simulink model "bh_DDR_component_model"  (R2019b)
settings: Solver=ode45  StartTime=0.0  StopTime=120  RelTol=1e-5  EnableMultiTasking=on
undefined symbols (not defined in the file): veh
libraries: simulink_extras x2
settings Model: Creator=sriramn  LastModifiedBy=Pierce
settings SolverCC: ZeroCrossAlgorithm=Adaptive
settings DataIOCC: LimitDataPoints=on  SaveFormat=Array  ReturnWorkspaceOutputs=off
settings OptimizationCC: LifeSpan=inf
settings DebuggingCC: AlgebraicLoopMsg=error  SolverPrmCheckMsg=warning  AllowSymbolicDim=off  SFUnexpectedBacktrackingDiag=warning  SFNoUnconditionalDefaultTransitionDiag=warning  SFExecutionAtInitializationDiag=none  ArithmeticOperatorsInVariantConditions=warning
settings HardwareCC: ProdBitPerPointer=32  ProdBitPerSizeT=32  ProdBitPerPtrDiffT=32  ProdLargestAtomicFloat=None  ProdIntDivRoundTo=Undefined  ProdEndianess=Unspecified  ProdWordSize=32  ProdHWDeviceType=32-bit Generic
settings ModelReferenceCC: PropagateSignalLabelsOutOfModel=off
settings SFSimCC: SimUseLocalCustomCode=off  CustomCodeUndefinedFunction=UseInterfaceOnly
settings RTWCC: RTWUseLocalCustomCode=off
settings CodeAppCC: StateflowObjectComments=on
settings GRTTargetCC: TargetLangStandard=C89/C90 (ANSI)  GeneratePreprocessorConditionals=Disable all
settings ConfigComp: CovMetricSettings=dw  CovHtmlReporting=on  CovSaveCumulativeToWorkspaceVar=on  CovSaveSingleToWorkspaceVar=on  CovExternalEMLEnable=off  CovSFcnEnable=off
settings SimscapeCC: SimscapeNormalizeSystem=off
settings ConfigurationSet: Description=SimMechanics 2G
settings ExplorerConfigSet: InternalSimMechanicsExplorerSettings="<ExplorerConfiguration><canonicalview>planar_xy</canonicalview><AnimationSetting><BasePlaybackSpeed>1.0</BasePlaybackSpeed><PlaybackSpeedFactor>1.0</PlaybackSpeedFactor></AnimationSetting><TilePanel><TileInfo><Tiles Columns=\"1\" Count=\"1\" Rows=\"1\"><Column Left=\"2\" Weight=\"1\"/><Column Left=\"1628\"/><Row Top=\"2\" Weight=\"1\"/><Row Top=\"1072\"/><Tile Height=\"1\" Width=\"1\" X=\"0\" Y=\"0\"/></Tiles></TileInfo><SceneInfo><SceneViewer><BGColor><R>0.60000002384185791</R><G>0.60000002384185791</G><B>0.60000002384185791</B></BGColor><Camera><Position><X>0.22951840878551699</X><Y>0.32651610611526627</Y><Z>-0.27215421354393321</Z></Position><Center><X>-0.15775714411666431</X><Y>-0.15462825985839526</Y><Z>0.065702552916005602</Z></Center><Up><X>-0.56030137557930915</X><Y>0.72817587161684794</Y><Z>0.39474329445726858</Z></Up><Left>-0.21481383955700509</Left><Right>0.21481383955700509</Right><Bottom>-0.27569784609469139</Bottom><Top>0.27569784609469139</Top></Camera></SceneViewer></SceneInfo></TilePanel></ExplorerConfiguration>"

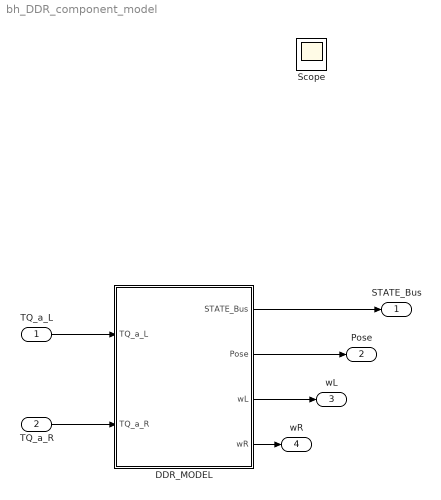
== system bh_DDR_component_model ==
  TQ_a_L : Inport
  TQ_a_R : Inport  Port=2
  DDR_MODEL : Subsystem  mask(EOM for differential drive robot){L=veh.L_half_axle, d=veh.d, m=veh.mass, I_veh=veh.Inertia, r=veh.wheel.r, m_w=veh.wheel.mass, I_w=veh.wheel.I, bR=veh.wheel.bR, bL=veh.wheel.bL, v_Cx_init=veh.states.init_vel_B_Cx, theta0_degs=0, theta0_dot_degs_per_sec=veh.states.init_theta_vel_deg, xy_G_init=[2,2]}
      mask prompts: L "Axle HALF length (L) separating wheels  (m)"; d "the offset (d) of Cg from axle (m)"; m "Total Vehicle mass (m) in (kg)"; I_veh "Total Vehicle Inertia (I_veh) in (kg.m^2)"; r "Radius (r) of driving wheels (m)"; m_w "Wheel mass (m_w) in (kg)"; I_w "Wheel and local shaft Inertia (Iw) in (kg.m^2)"; bR "RIGHT shaft viscous dampng (bR) in (N.m.sec/rad)"; bL "LEFT shaft viscous dampng (bR) in (N.m.sec/rad)"; v_Cx_init "Initial velocity vCx in the BODY  frame (m/sec)"; theta0_degs "Initial Theta position (degs)"; theta0_dot_degs_per_sec "Initial Theta velocity (degs/sec)"; xy_G_init "Initial (x,y) position in the {G}-frame (m)"
      mask help: Dynamic Model for a differential Drive robot.
      mask DialogControl Container10 Prompt: GEOMETRY
      mask DialogControl Container9 Prompt: INERTIA
      mask DialogControl Container12 Prompt: WHEELS
      mask DialogControl Control5 Prompt: We'll assume that the mass and inertia of the two wheels are the same, but we will let each wheel have different viscous damping.
      mask DialogControl Container6 Prompt: STATES
      mask Display: image(imread('bh_pics_veh_01.JPG'));
  STATE_Bus : Outport  OutDataTypeStr=Bus: BUS_DDR_state
  Pose : Outport  Port=2
  wL : Outport  Port=3
  wR : Outport  Port=4
  Scope : Scope
  wires:
  DDR_MODEL/1(STATE_Bus) -> STATE_Bus/1
  DDR_MODEL/2(Pose) -> Pose/1
  DDR_MODEL/3(wL) -> wL/1
  DDR_MODEL/4(wR) -> wR/1
  TQ_a_L/1 -> DDR_MODEL/1(TQ_a_L)
  TQ_a_R/1 -> DDR_MODEL/2(TQ_a_R)

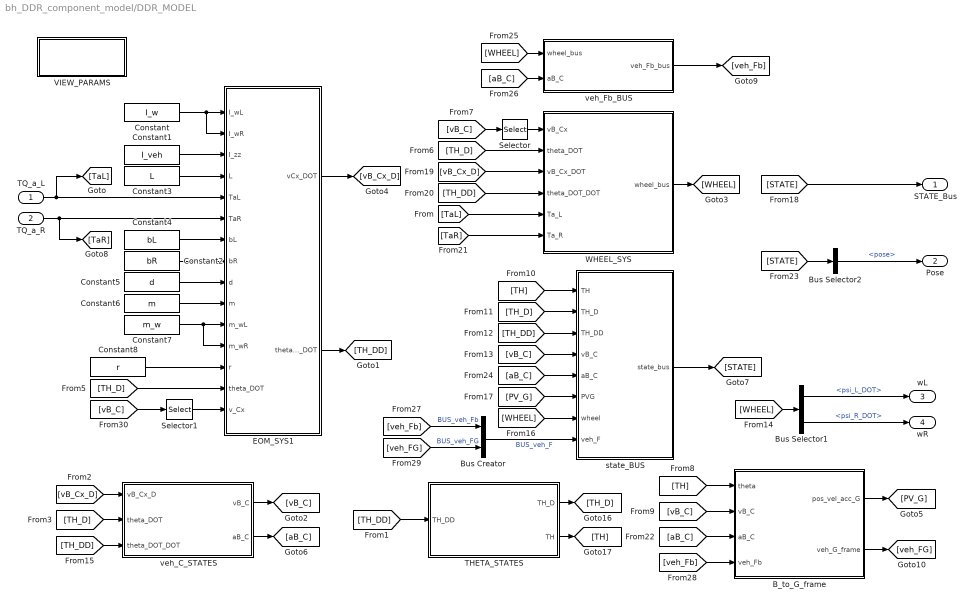
== system bh_DDR_component_model/DDR_MODEL ==
  TQ_a_L : Inport
  TQ_a_R : Inport  Port=2
  B_to_G_frame : Subsystem
  Bus Creator : BusCreator  Inputs=2
  Bus Selector1 : BusSelector  OutputSignals=BUS_wheel_vel.psi_L_DOT,BUS_wheel_vel.psi_R_DOT
  Bus Selector2 : BusSelector  OutputSignals=pose
  Constant : Constant  Value=I_w
  Constant1 : Constant  Value=I_veh
  Constant2 : Constant  Value=bR
  Constant3 : Constant  Value=L
  Constant4 : Constant  Value=bL
  Constant5 : Constant  Value=d
  Constant6 : Constant  Value=m
  Constant7 : Constant  Value=m_w
  Constant8 : Constant  Value=r
  EOM_SYS1 : MATLAB Function  TreatAsAtomicUnit=on
  Selector : Selector  InputPortWidth=2  IndexOptions=Index vector (dialog)  Indices=1  OutputSizes=1
  Selector1 : Selector  InputPortWidth=2  IndexOptions=Index vector (dialog)  Indices=1  OutputSizes=1
  THETA_STATES : Subsystem
  VIEW_PARAMS : Subsystem
  WHEEL_SYS : Subsystem
  state_BUS : Subsystem
  veh_C_STATES : Subsystem
  veh_Fb_BUS : Subsystem
  STATE_Bus : Outport
  Pose : Outport  Port=2
  wL : Outport  Port=3
  wR : Outport  Port=4
  wires:
  Constant1/1 -> EOM_SYS1/3(I_zz)
  Constant3/1 -> EOM_SYS1/4(L)
  Constant2/1 -> EOM_SYS1/8(bR)
  Constant4/1 -> EOM_SYS1/7(bL)
  Constant5/1 -> EOM_SYS1/9(d)
  Constant6/1 -> EOM_SYS1/10(m)
  Constant8/1 -> EOM_SYS1/13(r)
  TQ_a_L/1 -> EOM_SYS1/5(TaL), [TaL]
  TQ_a_R/1 -> EOM_SYS1/6(TaR), [TaR]
  [TH_DD] -> THETA_STATES/1(TH_DD)
  THETA_STATES/1(TH_D) -> [TH_D]
  THETA_STATES/2(TH) -> [TH]
  EOM_SYS1/2(theta_DOT_DOT) -> [TH_DD]
  [vB_Cx_D] -> veh_C_STATES/1(vB_Cx_D)
  EOM_SYS1/1(vCx_DOT) -> [vB_Cx_D]
  veh_C_STATES/1(vB_C) -> [vB_C]
  [TH_D] -> EOM_SYS1/14(theta_DOT)
  Selector1/1 -> EOM_SYS1/15(v_Cx)
  [vB_C] -> Selector/1
  [vB_C] -> B_to_G_frame/2(vB_C)
  [TH] -> B_to_G_frame/1(theta)
  B_to_G_frame/1(pos_vel_acc_G) -> [PV_G]
  [TH] -> state_BUS/1(TH)
  [TH_D] -> state_BUS/2(TH_D)
  [TH_DD] -> state_BUS/3(TH_DD)
  [WHEEL] -> state_BUS/7(wheel)
  [PV_G] -> state_BUS/6(PVG)
  state_BUS/1(state_bus) -> [STATE]
  [STATE] -> STATE_Bus/1
  [TH_D] -> WHEEL_SYS/2(theta_DOT)
  [vB_Cx_D] -> WHEEL_SYS/3(vB_Cx_DOT)
  [TH_DD] -> WHEEL_SYS/4(theta_DOT_DOT)
  WHEEL_SYS/1(wheel_bus) -> [WHEEL]
  [TaL] -> WHEEL_SYS/5(Ta_L)
  [TaR] -> WHEEL_SYS/6(Ta_R)
  [TH_D] -> veh_C_STATES/2(theta_DOT)
  Selector/1 -> WHEEL_SYS/1(vB_Cx)
  [vB_C] -> state_BUS/4(vB_C)
  [aB_C] -> state_BUS/5(aB_C)
  [TH_DD] -> veh_C_STATES/3(theta_DOT_DOT)
  veh_C_STATES/2(aB_C) -> [aB_C]
  [aB_C] -> B_to_G_frame/3(aB_C)
  [WHEEL] -> Bus Selector1/1
  Bus Selector1/1 -> wL/1  "<psi_L_DOT>"
  Bus Selector1/2 -> wR/1  "<psi_R_DOT>"
  [STATE] -> Bus Selector2/1
  Bus Selector2/1 -> Pose/1  "<pose>"
  [aB_C] -> veh_Fb_BUS/2(aB_C)
  [WHEEL] -> veh_Fb_BUS/1(wheel_bus)
  veh_Fb_BUS/1(veh_Fb_bus) -> [veh_Fb]
  [veh_Fb] -> B_to_G_frame/4(veh_Fb)
  B_to_G_frame/2(veh_G_frame) -> [veh_FG]
  [veh_Fb] -> Bus Creator/1  "BUS_veh_Fb"
  [veh_FG] -> Bus Creator/2  "BUS_veh_FG"
  Bus Creator/1 -> state_BUS/8(veh_F)  "BUS_veh_F"
  Constant/1 -> EOM_SYS1/2(I_wR), EOM_SYS1/1(I_wL)
  Constant7/1 -> EOM_SYS1/12(m_wR), EOM_SYS1/11(m_wL)
  [vB_C] -> Selector1/1

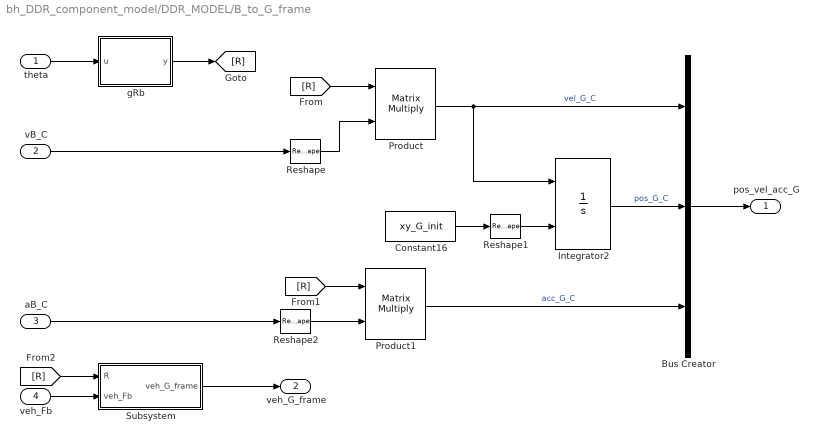
== system bh_DDR_component_model/DDR_MODEL/B_to_G_frame ==
  theta : Inport
  vB_C : Inport  Port=2
  aB_C : Inport  Port=3
  veh_Fb : Inport  Port=4
  Bus Creator : BusCreator  Inputs=3
  Constant16 : Constant  Value=xy_G_init
  Integrator2 : Integrator  InitialConditionSource=external
  Product : Product  Multiplication=Matrix(*)
  Product1 : Product  Multiplication=Matrix(*)
  Reshape : Reshape
  Reshape1 : Reshape
  Reshape2 : Reshape
  Subsystem : Subsystem
  gRb : MATLAB Function  TreatAsAtomicUnit=on
  pos_vel_acc_G : Outport
  veh_G_frame : Outport  Port=2
  wires:
  theta/1 -> gRb/1(u)
  Reshape/1 -> Product/2
  Product/1 -> Integrator2/1, Bus Creator/1  "vel_G_C"
  Constant16/1 -> Reshape1/1
  Integrator2/1 -> Bus Creator/2  "pos_G_C"
  Reshape1/1 -> Integrator2/2
  Bus Creator/1 -> pos_vel_acc_G/1
  vB_C/1 -> Reshape/1
  gRb/1(y) -> [R]
  [R] -> Product/1
  aB_C/1 -> Reshape2/1
  Reshape2/1 -> Product1/2
  [R] -> Product1/1
  Product1/1 -> Bus Creator/3  "acc_G_C"
  [R] -> Subsystem/1(R)
  veh_Fb/1 -> Subsystem/2(veh_Fb)
  Subsystem/1(veh_G_frame) -> veh_G_frame/1

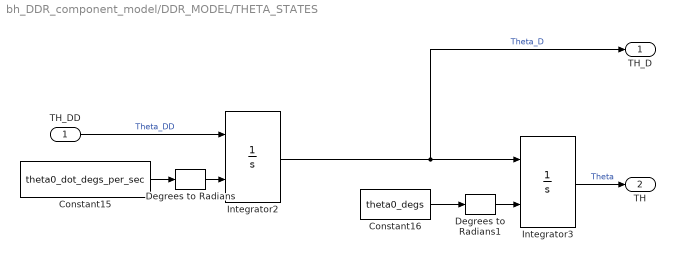
== system bh_DDR_component_model/DDR_MODEL/THETA_STATES ==
  TH_DD : Inport
  Constant15 : Constant  Value=theta0_dot_degs_per_sec
  Constant16 : Constant  Value=theta0_degs
  Degrees to Radians : simulink_extras/Transformations/Degrees to Radians
  Degrees to Radians1 : simulink_extras/Transformations/Degrees to Radians
  Integrator2 : Integrator  InitialConditionSource=external
  Integrator3 : Integrator  InitialConditionSource=external
  TH_D : Outport
  TH : Outport  Port=2
  wires:
  TH_DD/1 -> Integrator2/1  "Theta_DD"
  Integrator3/1 -> TH/1  "Theta"
  Integrator2/1 -> TH_D/1, Integrator3/1  "Theta_D"
  Degrees to Radians/1 -> Integrator2/2
  Degrees to Radians1/1 -> Integrator3/2
  Constant16/1 -> Degrees to Radians1/1
  Constant15/1 -> Degrees to Radians/1

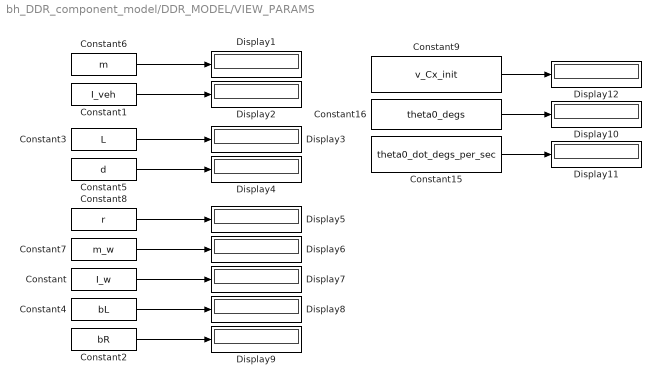
== system bh_DDR_component_model/DDR_MODEL/VIEW_PARAMS ==
  Constant : Constant  Value=I_w
  Constant1 : Constant  Value=I_veh
  Constant15 : Constant  Value=theta0_dot_degs_per_sec
  Constant16 : Constant  Value=theta0_degs
  Constant2 : Constant  Value=bR
  Constant3 : Constant  Value=L
  Constant4 : Constant  Value=bL
  Constant5 : Constant  Value=d
  Constant6 : Constant  Value=m
  Constant7 : Constant  Value=m_w
  Constant8 : Constant  Value=r
  Constant9 : Constant  Value=v_Cx_init
  Display{1..12} (12 alike) : Display
  wires:
  Constant6/1 -> Display1/1
  Constant1/1 -> Display2/1
  Constant5/1 -> Display4/1
  Constant3/1 -> Display3/1
  Constant7/1 -> Display6/1
  Constant8/1 -> Display5/1
  Constant/1 -> Display7/1
  Constant4/1 -> Display8/1
  Constant2/1 -> Display9/1
  Constant9/1 -> Display12/1
  Constant16/1 -> Display10/1
  Constant15/1 -> Display11/1

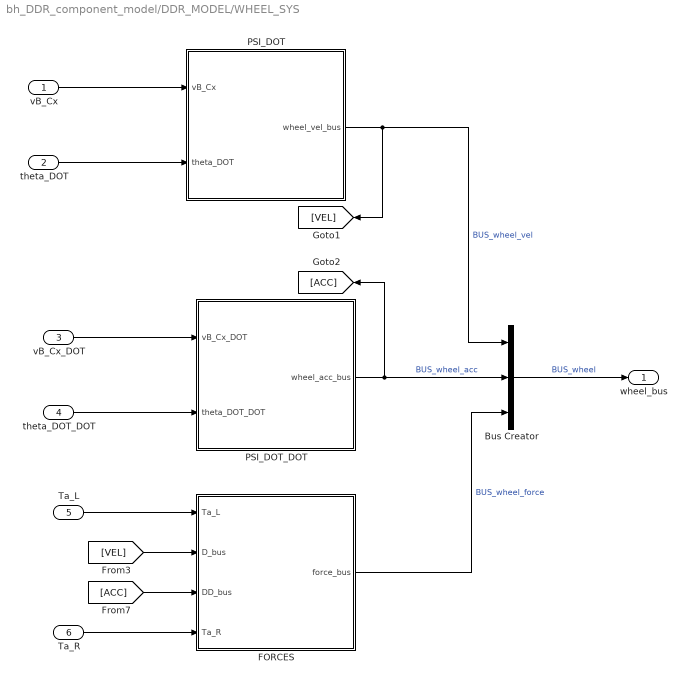
== system bh_DDR_component_model/DDR_MODEL/WHEEL_SYS ==
  vB_Cx : Inport
  theta_DOT : Inport  Port=2
  vB_Cx_DOT : Inport  Port=3
  theta_DOT_DOT : Inport  Port=4
  Ta_L : Inport  Port=5
  Ta_R : Inport  Port=6
  Bus Creator : BusCreator  Inputs=3
  FORCES : Subsystem
  PSI_DOT : Subsystem
  PSI_DOT_DOT : Subsystem
  wheel_bus : Outport
  wires:
  theta_DOT_DOT/1 -> PSI_DOT_DOT/2(theta_DOT_DOT)
  vB_Cx_DOT/1 -> PSI_DOT_DOT/1(vB_Cx_DOT)
  theta_DOT/1 -> PSI_DOT/2(theta_DOT)
  vB_Cx/1 -> PSI_DOT/1(vB_Cx)
  Bus Creator/1 -> wheel_bus/1  "BUS_wheel"
  PSI_DOT/1(wheel_vel_bus) -> [VEL], Bus Creator/1  "BUS_wheel_vel"
  PSI_DOT_DOT/1(wheel_acc_bus) -> Bus Creator/2, [ACC]  "BUS_wheel_acc"
  Ta_R/1 -> FORCES/4(Ta_R)
  Ta_L/1 -> FORCES/1(Ta_L)
  [ACC] -> FORCES/3(DD_bus)
  [VEL] -> FORCES/2(D_bus)
  FORCES/1(force_bus) -> Bus Creator/3  "BUS_wheel_force"

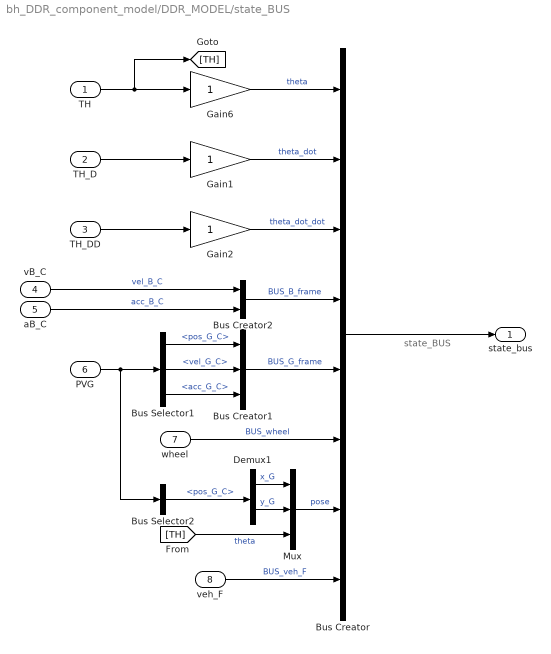
== system bh_DDR_component_model/DDR_MODEL/state_BUS ==
  note: state_BUS
  TH : Inport
  TH_D : Inport  Port=2
  TH_DD : Inport  Port=3
  vB_C : Inport  Port=4
  aB_C : Inport  Port=5
  PVG : Inport  Port=6
  wheel : Inport  Port=7
  veh_F : Inport  Port=8
  Bus Creator : BusCreator  Inputs=8
  Bus Creator1 : BusCreator  Inputs=3
  Bus Creator2 : BusCreator  Inputs=2
  Bus Selector1 : BusSelector  OutputSignals=pos_G_C,vel_G_C,acc_G_C
  Bus Selector2 : BusSelector  OutputSignals=pos_G_C
  Demux1 : Demux  Outputs=2
  Gain1 : Gain
  Gain2 : Gain
  Gain6 : Gain
  Mux : Mux  Inputs=3
  state_bus : Outport
  wires:
  Bus Creator/1 -> state_bus/1
  TH/1 -> [TH], Gain6/1
  TH_D/1 -> Gain1/1
  Gain6/1 -> Bus Creator/1  "theta"
  Gain1/1 -> Bus Creator/2  "theta_dot"
  TH_DD/1 -> Gain2/1
  Gain2/1 -> Bus Creator/3  "theta_dot_dot"
  vB_C/1 -> Bus Creator2/1  "vel_B_C"
  aB_C/1 -> Bus Creator2/2  "acc_B_C"
  PVG/1 -> Bus Selector2/1, Bus Selector1/1
  Bus Creator1/1 -> Bus Creator/5  "BUS_G_frame"
  wheel/1 -> Bus Creator/6  "BUS_wheel"
  Bus Creator2/1 -> Bus Creator/4  "BUS_B_frame"
  Bus Selector1/3 -> Bus Creator1/3  "<acc_G_C>"
  Bus Selector1/1 -> Bus Creator1/1  "<pos_G_C>"
  Bus Selector1/2 -> Bus Creator1/2  "<vel_G_C>"
  Mux/1 -> Bus Creator/7  "pose"
  Demux1/2 -> Mux/2  "y_G"
  Demux1/1 -> Mux/1  "x_G"
  [TH] -> Mux/3  "theta"
  Bus Selector2/1 -> Demux1/1  "<pos_G_C>"
  veh_F/1 -> Bus Creator/8  "BUS_veh_F"

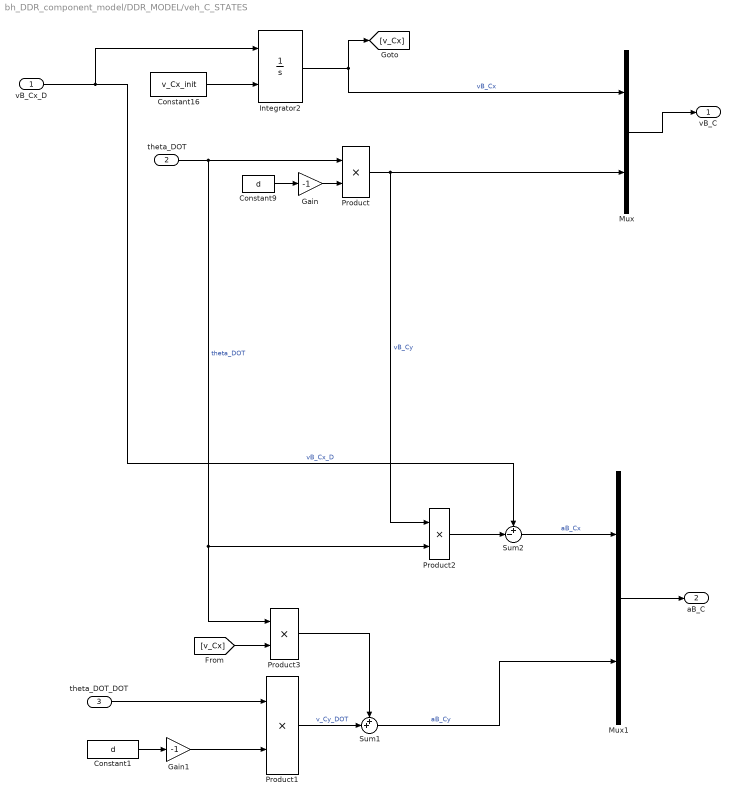
== system bh_DDR_component_model/DDR_MODEL/veh_C_STATES ==
  vB_Cx_D : Inport
  theta_DOT : Inport  Port=2
  theta_DOT_DOT : Inport  Port=3
  Constant1 : Constant  Value=d
  Constant16 : Constant  Value=v_Cx_init
  Constant9 : Constant  Value=d
  Gain : Gain  Gain=-1
  Gain1 : Gain  Gain=-1
  Integrator2 : Integrator  InitialConditionSource=external
  Mux : Mux  Inputs=2
  Mux1 : Mux  Inputs=2
  Product{,1..3} (4 alike) : Product
  Sum1 : Sum  Inputs=++|
  Sum2 : Sum  Inputs=+-|
  vB_C : Outport
  aB_C : Outport  Port=2
  wires:
  vB_Cx_D/1 -> Sum2/1, Integrator2/1  "vB_Cx_D"
  Constant16/1 -> Integrator2/2
  Integrator2/1 -> [v_Cx], Mux/1  "vB_Cx"
  theta_DOT/1 -> Product/1, Product3/1, Product2/2  "theta_DOT"
  Gain/1 -> Product/2
  Constant9/1 -> Gain/1
  Product/1 -> Product2/1, Mux/2  "vB_Cy"
  Mux/1 -> vB_C/1
  theta_DOT_DOT/1 -> Product1/1
  Gain1/1 -> Product1/2
  Constant1/1 -> Gain1/1
  Sum1/1 -> Mux1/2  "aB_Cy"
  Product2/1 -> Sum2/2
  Sum2/1 -> Mux1/1  "aB_Cx"
  Mux1/1 -> aB_C/1
  Product1/1 -> Sum1/2  "v_Cy_DOT"
  [v_Cx] -> Product3/2
  Product3/1 -> Sum1/1

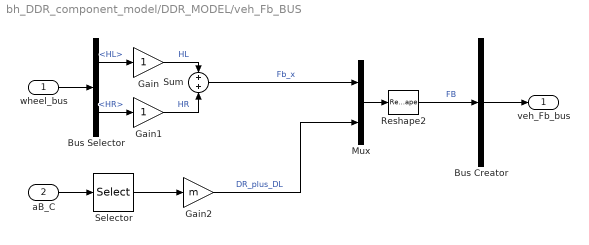
== system bh_DDR_component_model/DDR_MODEL/veh_Fb_BUS ==
  wheel_bus : Inport
  aB_C : Inport  Port=2
  Bus Creator : BusCreator  Inputs=1
  Bus Selector : BusSelector  OutputSignals=BUS_wheel_force.HL,BUS_wheel_force.HR
  Gain : Gain
  Gain1 : Gain
  Gain2 : Gain  Gain=m
  Mux : Mux  Inputs=2
  Reshape2 : Reshape
  Selector : Selector  InputPortWidth=2  IndexOptions=Index vector (dialog)  Indices=2  OutputSizes=1
  Sum : Sum  Inputs=+|+
  veh_Fb_bus : Outport
  wires:
  wheel_bus/1 -> Bus Selector/1
  Bus Selector/1 -> Gain/1  "<HL>"
  Bus Selector/2 -> Gain1/1  "<HR>"
  Gain/1 -> Sum/1  "HL"
  Gain1/1 -> Sum/2  "HR"
  Reshape2/1 -> Bus Creator/1  "FB"
  aB_C/1 -> Selector/1
  Selector/1 -> Gain2/1
  Sum/1 -> Mux/1  "Fb_x"
  Gain2/1 -> Mux/2  "DR_plus_DL"
  Mux/1 -> Reshape2/1
  Bus Creator/1 -> veh_Fb_bus/1

== system bh_DDR_component_model/DDR_MODEL/B_to_G_frame/Subsystem ==
  R : Inport
  veh_Fb : Inport  Port=2
  Bus Creator : BusCreator  Inputs=1
  Bus Selector : BusSelector  OutputSignals=FB
  Product1 : Product  Multiplication=Matrix(*)
  Reshape2 : Reshape
  veh_G_frame : Outport
  wires:
  Bus Selector/1 -> Reshape2/1  "<FB>"
  Reshape2/1 -> Product1/2
  R/1 -> Product1/1
  veh_Fb/1 -> Bus Selector/1
  Product1/1 -> Bus Creator/1  "FG"
  Bus Creator/1 -> veh_G_frame/1

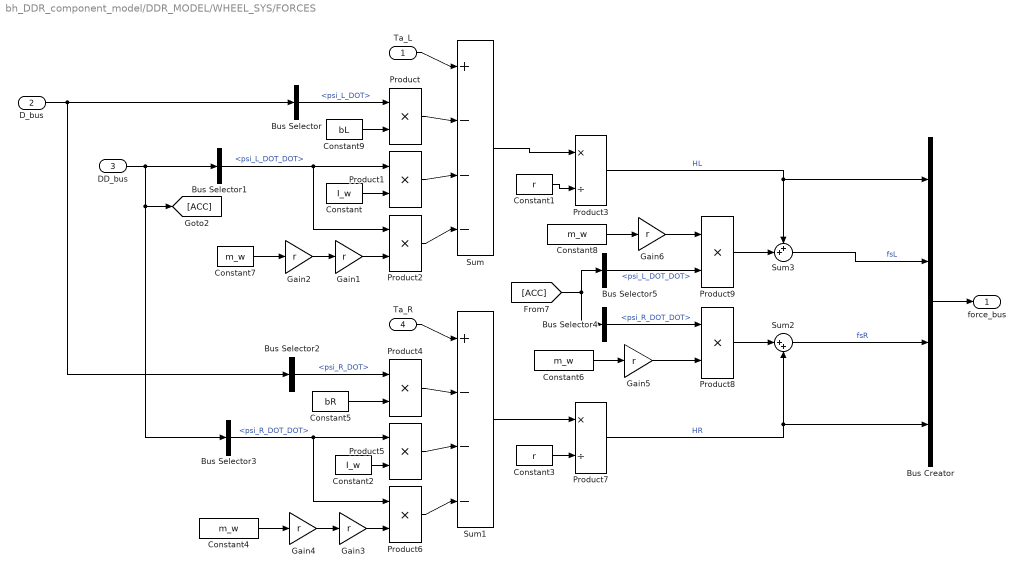
== system bh_DDR_component_model/DDR_MODEL/WHEEL_SYS/FORCES ==
  Ta_L : Inport
  D_bus : Inport  Port=2
  DD_bus : Inport  Port=3
  Ta_R : Inport  Port=4
  Bus Creator : BusCreator  Inputs=4
  Bus Selector : BusSelector  OutputSignals=psi_L_DOT
  Bus Selector1 : BusSelector  OutputSignals=psi_L_DOT_DOT
  Bus Selector2 : BusSelector  OutputSignals=psi_R_DOT
  Bus Selector3 : BusSelector  OutputSignals=psi_R_DOT_DOT
  Bus Selector4 : BusSelector  OutputSignals=psi_R_DOT_DOT
  Bus Selector5 : BusSelector  OutputSignals=psi_L_DOT_DOT
  Constant : Constant  Value=I_w
  Constant1 : Constant  Value=r
  Constant2 : Constant  Value=I_w
  Constant3 : Constant  Value=r
  Constant{4,6..8} (4 alike) : Constant  Value=m_w
  Constant5 : Constant  Value=bR
  Constant9 : Constant  Value=bL
  Gain{1..6} (6 alike) : Gain  Gain=r
  Product{,1..2,4..6,8..9} (8 alike) : Product
  Product3 : Product  Inputs=*/
  Product7 : Product  Inputs=*/
  Sum : Sum  Inputs=+|-|-|-
  Sum1 : Sum  Inputs=+|-|-|-
  Sum2 : Sum  Inputs=|++
  Sum3 : Sum  Inputs=++|
  force_bus : Outport
  wires:
  Constant9/1 -> Product/2
  Bus Selector/1 -> Product/1  "<psi_L_DOT>"
  Bus Selector1/1 -> Product2/1, Product1/1  "<psi_L_DOT_DOT>"
  Constant/1 -> Product1/2
  Constant7/1 -> Gain2/1
  Gain2/1 -> Gain1/1
  Gain1/1 -> Product2/2
  Product2/1 -> Sum/4
  Product1/1 -> Sum/3
  Product/1 -> Sum/2
  Constant1/1 -> Product3/2
  Sum/1 -> Product3/1
  Product3/1 -> Sum3/1, Bus Creator/1  "HL"
  D_bus/1 -> Bus Selector/1, Bus Selector2/1
  Constant5/1 -> Product4/2
  Bus Selector2/1 -> Product4/1  "<psi_R_DOT>"
  DD_bus/1 -> Bus Selector3/1, [ACC], Bus Selector1/1
  Bus Selector3/1 -> Product6/1, Product5/1  "<psi_R_DOT_DOT>"
  Constant2/1 -> Product5/2
  Constant4/1 -> Gain4/1
  Gain4/1 -> Gain3/1
  Gain3/1 -> Product6/2
  Ta_R/1 -> Sum1/1
  Product6/1 -> Sum1/4
  Product5/1 -> Sum1/3
  Product4/1 -> Sum1/2
  Constant3/1 -> Product7/2
  Sum1/1 -> Product7/1
  Product7/1 -> Sum2/2, Bus Creator/4  "HR"
  [ACC] -> Bus Selector4/1, Bus Selector5/1
  Constant6/1 -> Gain5/1
  Gain5/1 -> Product8/2
  Product8/1 -> Sum2/1
  Constant8/1 -> Gain6/1
  Gain6/1 -> Product9/1
  Bus Selector5/1 -> Product9/2  "<psi_L_DOT_DOT>"
  Product9/1 -> Sum3/2
  Sum3/1 -> Bus Creator/2  "fsL"
  Sum2/1 -> Bus Creator/3  "fsR"
  Ta_L/1 -> Sum/1
  Bus Creator/1 -> force_bus/1
  Bus Selector4/1 -> Product8/1  "<psi_R_DOT_DOT>"

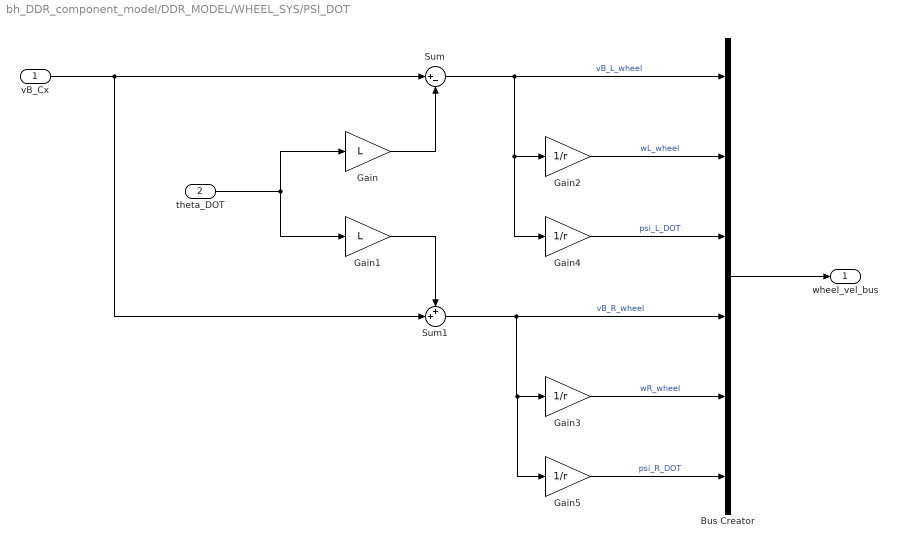
== system bh_DDR_component_model/DDR_MODEL/WHEEL_SYS/PSI_DOT ==
  vB_Cx : Inport
  theta_DOT : Inport  Port=2
  Bus Creator : BusCreator  Inputs=6
  Gain : Gain  Gain=L
  Gain1 : Gain  Gain=L
  Gain{2..5} (4 alike) : Gain  Gain=1/r
  Sum : Sum  Inputs=|+-
  Sum1 : Sum  Inputs=++|
  wheel_vel_bus : Outport
  wires:
  vB_Cx/1 -> Sum1/2, Sum/1
  theta_DOT/1 -> Gain/1, Gain1/1
  Gain/1 -> Sum/2
  Sum/1 -> Gain4/1, Gain2/1, Bus Creator/1  "vB_L_wheel"
  Gain1/1 -> Sum1/1
  Sum1/1 -> Bus Creator/4, Gain5/1, Gain3/1  "vB_R_wheel"
  Gain2/1 -> Bus Creator/2  "wL_wheel"
  Gain3/1 -> Bus Creator/5  "wR_wheel"
  Bus Creator/1 -> wheel_vel_bus/1
  Gain5/1 -> Bus Creator/6  "psi_R_DOT"
  Gain4/1 -> Bus Creator/3  "psi_L_DOT"

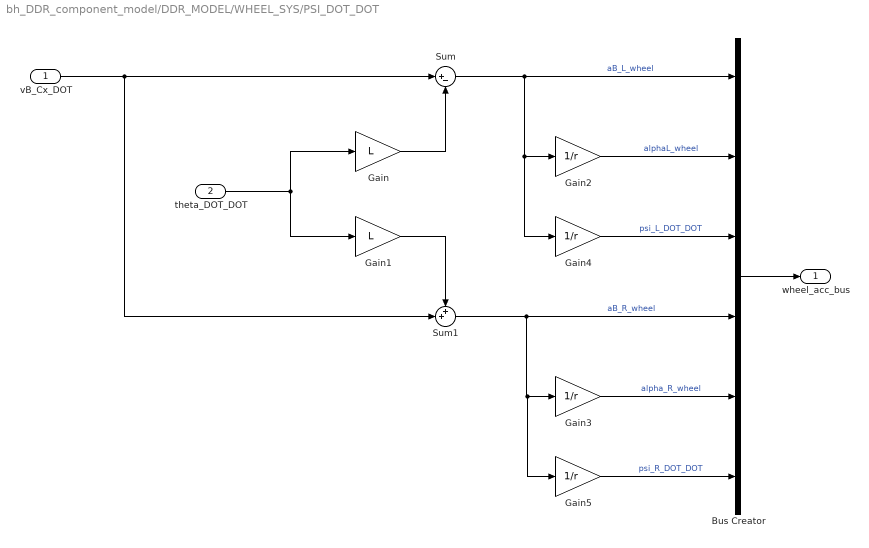
== system bh_DDR_component_model/DDR_MODEL/WHEEL_SYS/PSI_DOT_DOT ==
  vB_Cx_DOT : Inport
  theta_DOT_DOT : Inport  Port=2
  Bus Creator : BusCreator  Inputs=6
  Gain : Gain  Gain=L
  Gain1 : Gain  Gain=L
  Gain{2..5} (4 alike) : Gain  Gain=1/r
  Sum : Sum  Inputs=|+-
  Sum1 : Sum  Inputs=++|
  wheel_acc_bus : Outport
  wires:
  vB_Cx_DOT/1 -> Sum1/2, Sum/1
  theta_DOT_DOT/1 -> Gain/1, Gain1/1
  Gain/1 -> Sum/2
  Sum/1 -> Gain4/1, Gain2/1, Bus Creator/1  "aB_L_wheel"
  Gain1/1 -> Sum1/1
  Sum1/1 -> Bus Creator/4, Gain5/1, Gain3/1  "aB_R_wheel"
  Gain2/1 -> Bus Creator/2  "alphaL_wheel"
  Gain3/1 -> Bus Creator/5  "alpha_R_wheel"
  Bus Creator/1 -> wheel_acc_bus/1
  Gain5/1 -> Bus Creator/6  "psi_R_DOT_DOT"
  Gain4/1 -> Bus Creator/3  "psi_L_DOT_DOT"

== matlab function bh_DDR_component_model/DDR_MODEL/EOM_SYS1 ==
  data: I_wL input; vCx_DOT output; I_wR input; I_zz input; L input; TaL input; TaR input; bL input; bR input; d input; m input; m_wL input; m_wR input; r input; theta_DOT input; v_Cx input; theta_DOT_DOT output
function [vCx_DOT,theta_DOT_DOT] = EOM_SYS(I_wL,I_wR,I_zz,L,TaL,TaR,bL,bR,d,m,m_wL,m_wR,r,theta_DOT,v_Cx)
%#codegen

%    This function was generated by the Symbolic Math Toolbox version 7.1.
%    03-Dec-2016 14:01:57

t2 = r.^2;
t3 = t2.^2;
t4 = L.^2;
t5 = d.^2;
t6 = m.^2;
t7 = theta_DOT.^2;
t8 = I_wL.*I_wR.*t4.*4.0;
t9 = t3.*t5.*t6;
t10 = I_wL.*I_zz.*t2;
t11 = I_wR.*I_zz.*t2;
t12 = I_zz.*m.*t3;
t13 = I_zz.*m_wL.*t3;
t14 = I_zz.*m_wR.*t3;
t15 = I_wL.*m.*t2.*t4;
t16 = I_wR.*m.*t2.*t4;
t17 = I_wL.*m_wR.*t2.*t4.*4.0;
t18 = I_wR.*m_wL.*t2.*t4.*4.0;
t19 = I_wL.*m.*t2.*t5;
t20 = I_wR.*m.*t2.*t5;
t21 = m.*m_wL.*t3.*t4;
t22 = m.*m_wR.*t3.*t4;
t23 = m_wL.*m_wR.*t3.*t4.*4.0;
t24 = m.*m_wL.*t3.*t5;
t25 = m.*m_wR.*t3.*t5;
t26 = t8+t9+t10+t11+t12+t13+t14+t15+t16+t17+t18+t19+t20+t21+t22+t23+t24+t25;
t27 = 1.0./t26;
vCx_DOT = -t27.*(I_wR.*TaL.*r.*t4.*-2.0-I_zz.*TaL.*r.*t2-I_wL.*TaR.*r.*t4.*2.0-I_zz.*TaR.*r.*t2+I_wR.*bL.*t4.*v_Cx.*2.0+I_zz.*bL.*t2.*v_Cx+I_wL.*bR.*t4.*v_Cx.*2.0+I_zz.*bR.*t2.*v_Cx-I_wR.*L.*bL.*t4.*theta_DOT.*2.0-I_zz.*L.*bL.*t2.*theta_DOT+I_wL.*L.*bR.*t4.*theta_DOT.*2.0+I_zz.*L.*bR.*t2.*theta_DOT+I_zz.*d.*m.*t3.*t7-TaL.*m.*r.*t2.*t5-TaR.*m.*r.*t2.*t5-TaL.*m_wR.*r.*t2.*t4.*2.0-TaR.*m_wL.*r.*t2.*t4.*2.0+bL.*m.*t2.*t5.*v_Cx+bR.*m.*t2.*t5.*v_Cx+bL.*m_wR.*t2.*t4.*v_Cx.*2.0+bR.*m_wL.*t2.*t4.*v_Cx.*2.0+d.*t3.*t5.*t6.*t7+I_wL.*d.*m.*t2.*t4.*t7+I_wR.*d.*m.*t2.*t4.*t7-L.*bL.*m.*t2.*t5.*theta_DOT+L.*bR.*m.*t2.*t5.*theta_DOT-L.*bL.*m_wR.*t2.*t4.*theta_DOT.*2.0+L.*bR.*m_wL.*t2.*t4.*theta_DOT.*2.0+d.*m.*m_wL.*t3.*t4.*t7+d.*m.*m_wR.*t3.*t4.*t7-I_wL.*L.*d.*m.*t2.*theta_DOT.*v_Cx+I_wR.*L.*d.*m.*t2.*theta_DOT.*v_Cx-L.*d.*m.*m_wL.*t3.*theta_DOT.*v_Cx+L.*d.*m.*m_wR.*t3.*theta_DOT.*v_Cx);
if nargout > 1
    theta_DOT_DOT = -t27.*(I_wR.*L.*TaL.*r.*2.0-I_wL.*L.*TaR.*r.*2.0-I_wR.*L.*bL.*v_Cx.*2.0+I_wL.*L.*bR.*v_Cx.*2.0+I_wR.*bL.*t4.*theta_DOT.*2.0+I_wL.*bR.*t4.*theta_DOT.*2.0+L.*TaL.*m.*r.*t2-L.*TaR.*m.*r.*t2+L.*TaL.*m_wR.*r.*t2.*2.0-L.*TaR.*m_wL.*r.*t2.*2.0-L.*bL.*m.*t2.*v_Cx+L.*bR.*m.*t2.*v_Cx-L.*bL.*m_wR.*t2.*v_Cx.*2.0+L.*bR.*m_wL.*t2.*v_Cx.*2.0+bL.*m.*t2.*t4.*theta_DOT+bR.*m.*t2.*t4.*theta_DOT+bL.*m_wR.*t2.*t4.*theta_DOT.*2.0+bR.*m_wL.*t2.*t4.*theta_DOT.*2.0-d.*t3.*t6.*theta_DOT.*v_Cx+I_wL.*L.*d.*m.*t2.*t7-I_wR.*L.*d.*m.*t2.*t7+L.*d.*m.*m_wL.*t3.*t7-L.*d.*m.*m_wR.*t3.*t7-I_wL.*d.*m.*t2.*theta_DOT.*v_Cx-I_wR.*d.*m.*t2.*theta_DOT.*v_Cx-d.*m.*m_wL.*t3.*theta_DOT.*v_Cx-d.*m.*m_wR.*t3.*theta_DOT.*v_Cx);
end

== matlab function bh_DDR_component_model/DDR_MODEL/B_to_G_frame/gRb ==
  data: u input; y output
function y = fcn(u)

y = [ cos(u), -sin(u);
      sin(u),  cos(u) ];
  
end
